simulink model "sim"  (R2023b)
settings: Solver=VariableStepAuto  StartTime=0.0  StopTime=TSim  RelTol=1e-3
undefined symbols (not defined in the file): dampingCoeff, freqDist, initPos, initVel, magDist, mass, phaseDist, springCoeff
libraries: simulink x2
settings Model: Creator=uos  LastModifiedBy=uos

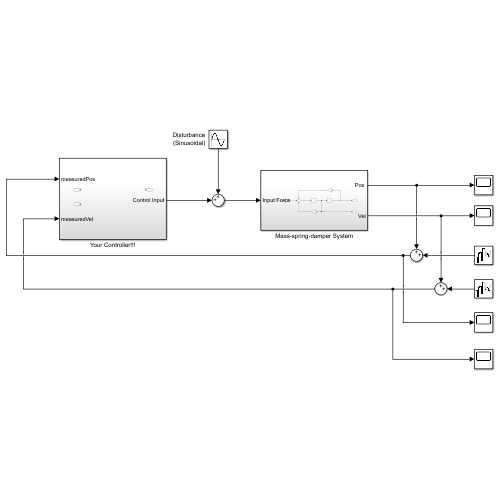
[thumbnail: Simulink's stored preview of the top-level diagram]
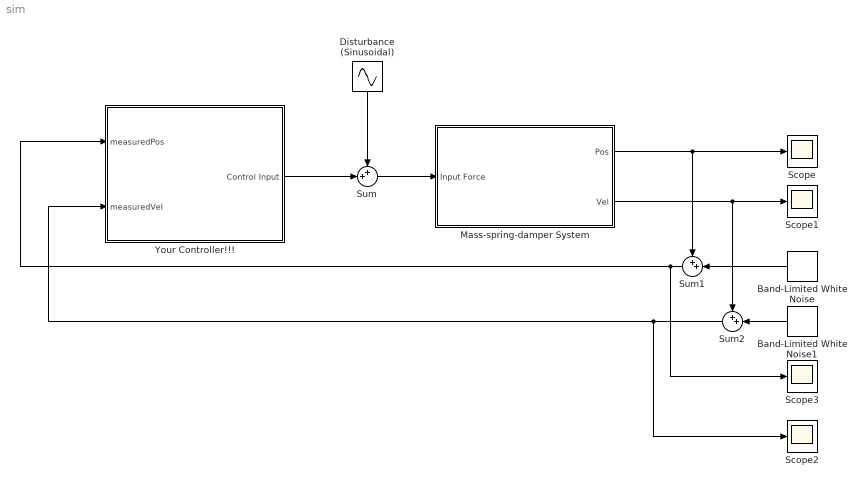
== system sim ==
  Band-Limited White Noise : simulink/Sources/Band-Limited White Noise  Cov=powerNoise  Ts=0.001  seed=[23341]
  Band-Limited White Noise1 : simulink/Sources/Band-Limited White Noise  Cov=powerNoise  Ts=0.001  seed=[23341]
  Disturbance (Sinusoidal) : Sin  Amplitude=magDist  Bias=phaseDist  Frequency=freqDist  SampleTime=0
  Mass-spring-damper System : Subsystem
  Scope{,1..3} (4 alike) : Scope
  Sum : Sum  Inputs=++|
  Sum1 : Sum  Inputs=++|
  Sum2 : Sum  Inputs=++|
  Your Controller!!! : Subsystem
  wires:
  Mass-spring-damper System/1("Pos ") -> Sum1/1, Scope/1
  Mass-spring-damper System/2(Vel) -> Sum2/1, Scope1/1
  Sum/1 -> Mass-spring-damper System/1("Input Force ")
  Band-Limited White Noise/1 -> Sum1/2
  Band-Limited White Noise1/1 -> Sum2/2
  Disturbance (Sinusoidal)/1 -> Sum/1
  Your Controller!!!/1(Control Input) -> Sum/2
  Sum1/1 -> Scope3/1, Your Controller!!!/1(measuredPos)
  Sum2/1 -> Scope2/1, Your Controller!!!/2(measuredVel)

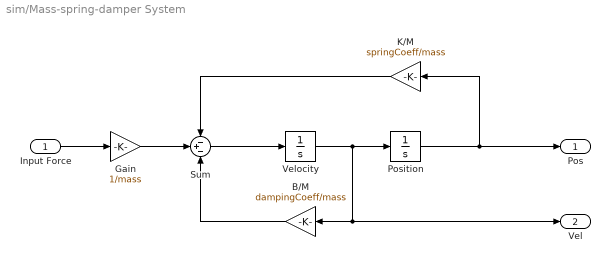
== system sim/Mass-spring-damper System ==
  "Input Force " : Inport
  B/M : Gain  Gain=dampingCoeff/mass
  Gain : Gain  Gain=1/mass
  K/M : Gain  Gain=springCoeff/mass
  Position : Integrator  InitialCondition=initPos
  Sum : Sum  Inputs=-+-
  Velocity : Integrator  InitialCondition=initVel
  "Pos " : Outport
  Vel : Outport  Port=2
  wires:
  Velocity/1 -> Vel/1, B/M/1, Position/1
  Gain/1 -> Sum/2
  "Input Force "/1 -> Gain/1
  Position/1 -> "Pos "/1, K/M/1
  K/M/1 -> Sum/1
  B/M/1 -> Sum/3
  Sum/1 -> Velocity/1

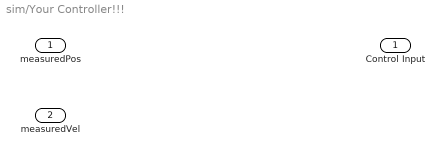
== system sim/Your Controller!!! ==
  measuredPos : Inport
  measuredVel : Inport  Port=2
  Control Input : Outport
